simulink library "sm_trackV_lib_chain_segment"  (R2026a)
settings: Solver=VariableStepAuto
undefined symbols (not defined in the file): Excv, X, Y, Z
libraries: sm_lib x43, $bdroot x10
(part 2 of 2)

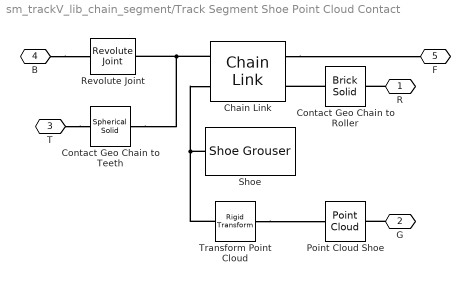
== system sm_trackV_lib_chain_segment/Track Segment Shoe Point Cloud Contact ==
  Chain Link : $bdroot/Chain Link  chain_wid=chain_wid  chain_seg_m=chain_seg_m  chain_seg_cg=chain_seg_cg  chain_seg_moi=chain_seg_moi  chain_seg_poi=chain_seg_poi  plate_h=plate_h  plate_xc=plate_xc  plate_thk=plate_thk  pin_sep=pin_sep  plate_ang=plate_ang  plate_clr=plate_clr  plate_opc=plate_opc  pin_len=pin_len  pin_rad=pin_rad  pin_clr=pin_clr  pin_opc=pin_opc
  Contact Geo Chain to Roller : sm_lib/Body Elements/Brick Solid  BrickDimensions=[pin_sep plate_h chain_wid/2]  BrickDimensionsUnits=m  ExportEntireGeometry=on  InertiaType=CalculateFromGeometry  BasedOnType=Density  Density=0  DensityUnits=kg/m^3  Mass=1  MassUnits=kg  CenterOfMass=[0 0 0]  CenterOfMassUnits=m  MomentsOfInertia=[1 1 1]  MomentsOfInertiaUnits=kg*m^2  ProductsOfInertia=[0 0 0]  ProductsOfInertiaUnits=kg*m^2  GraphicType=FromGeometry  MarkerShape=Sphere  MarkerSize=10  GraphicVisPropType=SimpleVisualProperties  GraphicDiffuseColor=chain_to_roller_clr  GraphicOpacity=chain_to_roller_opc  GraphicSpecularColor=[0.5 0.5 0.5 1.0]  GraphicAmbientColor=[0.15 0.15 0.15 1.0]  GraphicEmissiveColor=[0.0 0.0 0.0 1.0]  GraphicShininess=75  DoExposeReferenceFrame=on  SerializedFrames=<Frames/>
  Contact Geo Chain to Teeth : sm_lib/Body Elements/Spherical Solid  SphereRadius=pin_rad  SphereRadiusUnits=m  ExportEntireGeometry=on  InertiaType=CalculateFromGeometry  BasedOnType=Density  Density=0  DensityUnits=kg/m^3  Mass=1  MassUnits=kg  CenterOfMass=[0 0 0]  CenterOfMassUnits=m  MomentsOfInertia=[1 1 1]  MomentsOfInertiaUnits=kg*m^2  ProductsOfInertia=[0 0 0]  ProductsOfInertiaUnits=kg*m^2  GraphicType=FromGeometry  MarkerShape=Sphere  MarkerSize=10  GraphicVisPropType=SimpleVisualProperties  GraphicDiffuseColor=chain_to_teeth_clr  GraphicOpacity=chain_to_teeth_opc  GraphicSpecularColor=[0.5 0.5 0.5 1.0]  GraphicAmbientColor=[0.15 0.15 0.15 1.0]  GraphicEmissiveColor=[0.0 0.0 0.0 1.0]  GraphicShininess=75  DoExposeReferenceFrame=on  SerializedFrames=<Frames/>
  Point Cloud Shoe : sm_lib/Curves and Surfaces/Point Cloud  CoordinatesMatrix=ptcld_shoe  CoordinatesMatrixUnits=m  GraphicType=MarkerCloud  GraphicSphereRadius=ptcld_shoe_rad  GraphicSphereRadiusUnits=m  GraphicVisPropType=SimpleVisualProperties  GraphicDiffuseColor=ptcld_shoe_clr  GraphicOpacity=ptcld_shoe_opc  GraphicSpecularColor=[0.5 0.5 0.5 1.0]  GraphicAmbientColor=[0.15 0.15 0.15 1.0]  GraphicEmissiveColor=[0.0 0.0 0.0 1.0]  GraphicShininess=75
  Revolute Joint : sm_lib/Joints/Revolute Joint  JointMode=Normal  CompositeWrenchDir=FollowerOnBase  CompositeWrenchFrame=BaseFrame  SenseConstraintForce=off  SenseConstraintTorque=off  SenseTotalForce=off  SenseTotalTorque=off  PositionTargetSpecify=on  PositionTargetPriority=High  PositionTargetValue=PositionTargetValue  PositionTargetValueUnits=deg  VelocityTargetSpecify=off  VelocityTargetPriority=High  VelocityTargetValue=0  VelocityTargetValueUnits=deg/s  EquilibriumPosition=0  EquilibriumPositionUnits=deg  SpringStiffness=0  SpringStiffnessUnits=N*m/deg  DampingCoefficient=DampingCoefficient  DampingCoefficientUnits=N*m/(deg/s)  LowerLimitSpecify=off  LowerLimitBound=-10  LowerLimitBoundUnits=deg  LowerLimitStiffness=1e2  LowerLimitStiffnessUnits=N*m/deg  LowerLimitDamping=10  LowerLimitDampingUnits=N*m/(deg/s)  LowerLimitTransitionRegionWidth=0.1  LowerLimitTransitionRegionWidthUnits=deg  UpperLimitSpecify=off  UpperLimitBound=65  UpperLimitBoundUnits=deg  UpperLimitStiffness=1e2  UpperLimitStiffnessUnits=N*m/deg  UpperLimitDamping=10  UpperLimitDampingUnits=N*m/(deg/s)  UpperLimitTransitionRegionWidth=0.1  UpperLimitTransitionRegionWidthUnits=deg  TorqueActuationMode=NoTorque  MotionActuationMode=ComputedMotion  SensePosition=off  SenseVelocity=off  SenseAcceleration=off  SenseTorqueForce=off  SenseLowerLimitTorqueForce=off  SenseUpperLimitTorqueForce=off
  Shoe : $bdroot/Shoe Grouser  shoe_xc=shoe_xc  shoe_w=shoe_w  shoe_m=shoe_m  shoe_cg=shoe_cg  shoe_moi=shoe_moi  shoe_poi=shoe_poi  shoe_clr=shoe_clr  shoe_opc=shoe_opc
      settings: LibrarySourceBlock=sm_chain_drive_lib/Shoe
  Transform Point Cloud : sm_lib/Frames and Transforms/Rigid Transform  RotationMethod=StandardAxis  FollAlignAxisA=+X  BaseAlignAxisA=+Y  FollAlignAxisB=+Y  BaseAlignAxisB=+Z  RotationStandardAxis=+Y  RotationAngle=180  RotationAngleUnits=deg  RotationArbitraryAxis=[0 0 1]  RotationSequenceAxes=FollowerAxes  RotationSequence=XYX  RotationSequenceAngles=[0 0 0]  RotationSequenceAnglesUnits=deg  RotationMatrix=[1 0 0; 0 1 0; 0 0 1]  Quaternion=[1 0 0 0]  TranslationMethod=None  TranslationCartesianOffset=[0 0 0]  TranslationCartesianOffsetUnits=m  TranslationStandardAxis=-Y  TranslationStandardOffset=0  TranslationStandardOffsetUnits=m  TranslationROffset=0  TranslationROffsetUnits=m  TranslationThetaOffset=0  TranslationThetaOffsetUnits=deg  TranslationZOffset=0  TranslationZOffsetUnits=m
  R : PMIOPort  Side=Right
  G : PMIOPort  Port=2  Side=Right
  T : PMIOPort  Port=3  Side=Right
  B : PMIOPort  Port=4  Side=Left
  F : PMIOPort  Port=5  Side=Left
  connections:
  Transform Point Cloud/RConn1 -- Point Cloud Shoe/LConn1
  Contact Geo Chain to Teeth/RConn1 -- Chain Link/RConn1 -- Revolute Joint/LConn1
  Shoe/RConn1 -- Transform Point Cloud/LConn1 -- Chain Link/RConn2
  B/RConn1 -- Revolute Joint/RConn1
  G/RConn1 -- Point Cloud Shoe/RConn1
  T/RConn1 -- Contact Geo Chain to Teeth/LConn1
  Contact Geo Chain to Roller/RConn1 -- Chain Link/LConn2
  R/RConn1 -- Contact Geo Chain to Roller/LConn1
  Chain Link/LConn1 -- F/RConn1

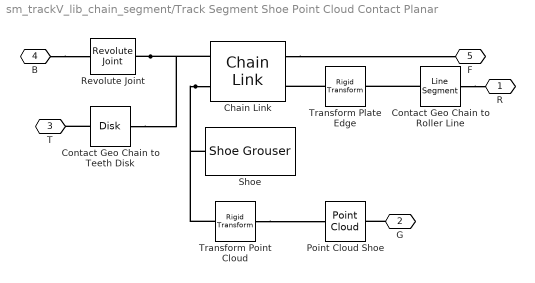
== system sm_trackV_lib_chain_segment/Track Segment Shoe Point Cloud Contact Planar ==
  Chain Link : $bdroot/Chain Link  chain_wid=chain_wid  chain_seg_m=chain_seg_m  chain_seg_cg=chain_seg_cg  chain_seg_moi=chain_seg_moi  chain_seg_poi=chain_seg_poi  plate_h=plate_h  plate_xc=plate_xc  plate_thk=plate_thk  pin_sep=pin_sep  plate_ang=plate_ang  plate_clr=plate_clr  plate_opc=plate_opc  pin_len=pin_len  pin_rad=pin_rad  pin_clr=pin_clr  pin_opc=pin_opc
  Contact Geo Chain to Roller Line : sm_lib/Curves and Surfaces/Line Segment  Length=pin_sep  LengthUnits=m  GraphicType=FromGeometry  GraphicVisPropType=SimpleVisualProperties  GraphicDiffuseColor=chain_to_roller_clr  GraphicOpacity=chain_to_roller_opc  GraphicSpecularColor=[0.5 0.5 0.5 1.0]  GraphicAmbientColor=[0.15 0.15 0.15 1.0]  GraphicEmissiveColor=[0.0 0.0 0.0 1.0]  GraphicShininess=75
  Contact Geo Chain to Teeth Disk : sm_lib/Curves and Surfaces/Disk  Radius=pin_rad  RadiusUnits=m  GraphicType=FromGeometry  GraphicVisPropType=SimpleVisualProperties  GraphicDiffuseColor=chain_to_teeth_clr  GraphicOpacity=chain_to_teeth_opc  GraphicSpecularColor=[0.5 0.5 0.5 1.0]  GraphicAmbientColor=[0.15 0.15 0.15 1.0]  GraphicEmissiveColor=[0.0 0.0 0.0 1.0]  GraphicShininess=75
  Point Cloud Shoe : sm_lib/Curves and Surfaces/Point Cloud  CoordinatesMatrix=ptcld_shoe  CoordinatesMatrixUnits=m  GraphicType=MarkerCloud  GraphicSphereRadius=ptcld_shoe_rad  GraphicSphereRadiusUnits=m  GraphicVisPropType=SimpleVisualProperties  GraphicDiffuseColor=ptcld_shoe_clr  GraphicOpacity=ptcld_shoe_opc  GraphicSpecularColor=[0.5 0.5 0.5 1.0]  GraphicAmbientColor=[0.15 0.15 0.15 1.0]  GraphicEmissiveColor=[0.0 0.0 0.0 1.0]  GraphicShininess=75
  Revolute Joint : sm_lib/Joints/Revolute Joint  JointMode=Normal  CompositeWrenchDir=FollowerOnBase  CompositeWrenchFrame=BaseFrame  SenseConstraintForce=off  SenseConstraintTorque=off  SenseTotalForce=off  SenseTotalTorque=off  PositionTargetSpecify=on  PositionTargetPriority=High  PositionTargetValue=PositionTargetValue  PositionTargetValueUnits=deg  VelocityTargetSpecify=off  VelocityTargetPriority=High  VelocityTargetValue=0  VelocityTargetValueUnits=deg/s  EquilibriumPosition=0  EquilibriumPositionUnits=deg  SpringStiffness=0  SpringStiffnessUnits=N*m/deg  DampingCoefficient=DampingCoefficient  DampingCoefficientUnits=N*m/(deg/s)  LowerLimitSpecify=off  LowerLimitBound=-10  LowerLimitBoundUnits=deg  LowerLimitStiffness=1e2  LowerLimitStiffnessUnits=N*m/deg  LowerLimitDamping=10  LowerLimitDampingUnits=N*m/(deg/s)  LowerLimitTransitionRegionWidth=0.1  LowerLimitTransitionRegionWidthUnits=deg  UpperLimitSpecify=off  UpperLimitBound=65  UpperLimitBoundUnits=deg  UpperLimitStiffness=1e2  UpperLimitStiffnessUnits=N*m/deg  UpperLimitDamping=10  UpperLimitDampingUnits=N*m/(deg/s)  UpperLimitTransitionRegionWidth=0.1  UpperLimitTransitionRegionWidthUnits=deg  TorqueActuationMode=NoTorque  MotionActuationMode=ComputedMotion  SensePosition=off  SenseVelocity=off  SenseAcceleration=off  SenseTorqueForce=off  SenseLowerLimitTorqueForce=off  SenseUpperLimitTorqueForce=off
  Shoe : $bdroot/Shoe Grouser  shoe_xc=shoe_xc  shoe_w=shoe_w  shoe_m=shoe_m  shoe_cg=shoe_cg  shoe_moi=shoe_moi  shoe_poi=shoe_poi  shoe_clr=shoe_clr  shoe_opc=shoe_opc
      settings: LibrarySourceBlock=sm_chain_drive_lib/Shoe
  Transform Plate Edge : sm_lib/Frames and Transforms/Rigid Transform  RotationMethod=None  FollAlignAxisA=+X  BaseAlignAxisA=+Y  FollAlignAxisB=+Y  BaseAlignAxisB=+Z  RotationStandardAxis=+Z  RotationAngle=0.0  RotationAngleUnits=deg  RotationArbitraryAxis=[0 0 1]  RotationSequenceAxes=FollowerAxes  RotationSequence=XYX  RotationSequenceAngles=[0 0 0]  RotationSequenceAnglesUnits=deg  RotationMatrix=[1 0 0; 0 1 0; 0 0 1]  Quaternion=[1 0 0 0]  TranslationMethod=StandardAxis  TranslationCartesianOffset=[0 0 0]  TranslationCartesianOffsetUnits=m  TranslationStandardAxis=+Y  TranslationStandardOffset=plate_h/2  TranslationStandardOffsetUnits=m  TranslationROffset=0  TranslationROffsetUnits=m  TranslationThetaOffset=0  TranslationThetaOffsetUnits=deg  TranslationZOffset=0  TranslationZOffsetUnits=m
  Transform Point Cloud : sm_lib/Frames and Transforms/Rigid Transform  RotationMethod=StandardAxis  FollAlignAxisA=+X  BaseAlignAxisA=+Y  FollAlignAxisB=+Y  BaseAlignAxisB=+Z  RotationStandardAxis=+Y  RotationAngle=180  RotationAngleUnits=deg  RotationArbitraryAxis=[0 0 1]  RotationSequenceAxes=FollowerAxes  RotationSequence=XYX  RotationSequenceAngles=[0 0 0]  RotationSequenceAnglesUnits=deg  RotationMatrix=[1 0 0; 0 1 0; 0 0 1]  Quaternion=[1 0 0 0]  TranslationMethod=None  TranslationCartesianOffset=[0 0 0]  TranslationCartesianOffsetUnits=m  TranslationStandardAxis=-Y  TranslationStandardOffset=0  TranslationStandardOffsetUnits=m  TranslationROffset=0  TranslationROffsetUnits=m  TranslationThetaOffset=0  TranslationThetaOffsetUnits=deg  TranslationZOffset=0  TranslationZOffsetUnits=m
  R : PMIOPort  Side=Right
  G : PMIOPort  Port=2  Side=Right
  T : PMIOPort  Port=3  Side=Right
  B : PMIOPort  Port=4  Side=Left
  F : PMIOPort  Port=5  Side=Left
  connections:
  Contact Geo Chain to Roller Line/LConn1 -- Transform Plate Edge/RConn1
  Chain Link/LConn1 -- F/RConn1
  Contact Geo Chain to Roller Line/RConn1 -- R/RConn1
  Transform Plate Edge/LConn1 -- Chain Link/LConn2
  Contact Geo Chain to Teeth Disk/RConn1 -- T/RConn1
  G/RConn1 -- Point Cloud Shoe/RConn1
  B/RConn1 -- Revolute Joint/RConn1
  Chain Link/RConn2 -- Transform Point Cloud/LConn1 -- Shoe/RConn1
  Revolute Joint/LConn1 -- Contact Geo Chain to Teeth Disk/LConn1 -- Chain Link/RConn1
  Transform Point Cloud/RConn1 -- Point Cloud Shoe/LConn1

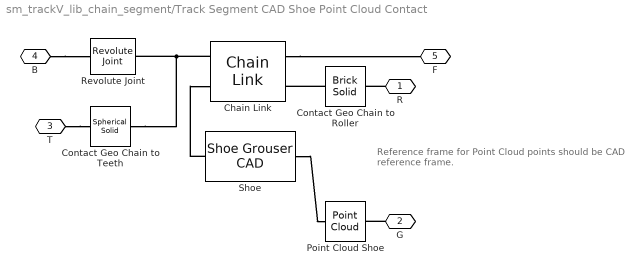
== system sm_trackV_lib_chain_segment/Track Segment CAD Shoe Point Cloud Contact ==
  note: Reference frame for Point Cloud points should be CAD reference frame.
  Chain Link : $bdroot/Chain Link  chain_wid=chain_wid  chain_seg_m=chain_seg_m  chain_seg_cg=chain_seg_cg  chain_seg_moi=chain_seg_moi  chain_seg_poi=chain_seg_poi  plate_h=plate_h  plate_xc=plate_xc  plate_thk=plate_thk  pin_sep=pin_sep  plate_ang=plate_ang  plate_clr=plate_clr  plate_opc=plate_opc  pin_len=pin_len  pin_rad=pin_rad  pin_clr=pin_clr  pin_opc=pin_opc
  Contact Geo Chain to Roller : sm_lib/Body Elements/Brick Solid  BrickDimensions=[pin_sep plate_h chain_wid/2]  BrickDimensionsUnits=m  ExportEntireGeometry=on  InertiaType=CalculateFromGeometry  BasedOnType=Density  Density=0  DensityUnits=kg/m^3  Mass=1  MassUnits=kg  CenterOfMass=[0 0 0]  CenterOfMassUnits=m  MomentsOfInertia=[1 1 1]  MomentsOfInertiaUnits=kg*m^2  ProductsOfInertia=[0 0 0]  ProductsOfInertiaUnits=kg*m^2  GraphicType=FromGeometry  MarkerShape=Sphere  MarkerSize=10  GraphicVisPropType=SimpleVisualProperties  GraphicDiffuseColor=chain_to_roller_clr  GraphicOpacity=chain_to_roller_opc  GraphicSpecularColor=[0.5 0.5 0.5 1.0]  GraphicAmbientColor=[0.15 0.15 0.15 1.0]  GraphicEmissiveColor=[0.0 0.0 0.0 1.0]  GraphicShininess=75  DoExposeReferenceFrame=on  SerializedFrames=<Frames/>
  Contact Geo Chain to Teeth : sm_lib/Body Elements/Spherical Solid  SphereRadius=pin_rad  SphereRadiusUnits=m  ExportEntireGeometry=on  InertiaType=CalculateFromGeometry  BasedOnType=Density  Density=0  DensityUnits=kg/m^3  Mass=1  MassUnits=kg  CenterOfMass=[0 0 0]  CenterOfMassUnits=m  MomentsOfInertia=[1 1 1]  MomentsOfInertiaUnits=kg*m^2  ProductsOfInertia=[0 0 0]  ProductsOfInertiaUnits=kg*m^2  GraphicType=FromGeometry  MarkerShape=Sphere  MarkerSize=10  GraphicVisPropType=SimpleVisualProperties  GraphicDiffuseColor=chain_to_teeth_clr  GraphicOpacity=chain_to_teeth_opc  GraphicSpecularColor=[0.5 0.5 0.5 1.0]  GraphicAmbientColor=[0.15 0.15 0.15 1.0]  GraphicEmissiveColor=[0.0 0.0 0.0 1.0]  GraphicShininess=75  DoExposeReferenceFrame=on  SerializedFrames=<Frames/>
  Point Cloud Shoe : sm_lib/Curves and Surfaces/Point Cloud  CoordinatesMatrix=ptcld_shoe  CoordinatesMatrixUnits=m  GraphicType=MarkerCloud  GraphicSphereRadius=ptcld_shoe_rad  GraphicSphereRadiusUnits=m  GraphicVisPropType=SimpleVisualProperties  GraphicDiffuseColor=ptcld_shoe_clr  GraphicOpacity=ptcld_shoe_opc  GraphicSpecularColor=[0.5 0.5 0.5 1.0]  GraphicAmbientColor=[0.15 0.15 0.15 1.0]  GraphicEmissiveColor=[0.0 0.0 0.0 1.0]  GraphicShininess=75
  Revolute Joint : sm_lib/Joints/Revolute Joint  JointMode=Normal  CompositeWrenchDir=FollowerOnBase  CompositeWrenchFrame=BaseFrame  SenseConstraintForce=off  SenseConstraintTorque=off  SenseTotalForce=off  SenseTotalTorque=off  PositionTargetSpecify=on  PositionTargetPriority=High  PositionTargetValue=PositionTargetValue  PositionTargetValueUnits=deg  VelocityTargetSpecify=off  VelocityTargetPriority=High  VelocityTargetValue=0  VelocityTargetValueUnits=deg/s  EquilibriumPosition=0  EquilibriumPositionUnits=deg  SpringStiffness=0  SpringStiffnessUnits=N*m/deg  DampingCoefficient=DampingCoefficient  DampingCoefficientUnits=N*m/(deg/s)  LowerLimitSpecify=off  LowerLimitBound=-10  LowerLimitBoundUnits=deg  LowerLimitStiffness=1e2  LowerLimitStiffnessUnits=N*m/deg  LowerLimitDamping=10  LowerLimitDampingUnits=N*m/(deg/s)  LowerLimitTransitionRegionWidth=0.1  LowerLimitTransitionRegionWidthUnits=deg  UpperLimitSpecify=off  UpperLimitBound=65  UpperLimitBoundUnits=deg  UpperLimitStiffness=1e2  UpperLimitStiffnessUnits=N*m/deg  UpperLimitDamping=10  UpperLimitDampingUnits=N*m/(deg/s)  UpperLimitTransitionRegionWidth=0.1  UpperLimitTransitionRegionWidthUnits=deg  TorqueActuationMode=NoTorque  MotionActuationMode=ComputedMotion  SensePosition=off  SenseVelocity=off  SenseAcceleration=off  SenseTorqueForce=off  SenseLowerLimitTorqueForce=off  SenseUpperLimitTorqueForce=off
  Shoe : $bdroot/Shoe Grouser CAD  shoe_xc=shoe_xc  shoe_w=shoe_w  shoe_m=shoe_m  shoe_cg=shoe_cg  shoe_moi=shoe_moi  shoe_poi=shoe_poi  shoe_clr=shoe_clr  shoe_opc=shoe_opc
  R : PMIOPort  Side=Right
  G : PMIOPort  Port=2  Side=Right
  T : PMIOPort  Port=3  Side=Right
  B : PMIOPort  Port=4  Side=Left
  F : PMIOPort  Port=5  Side=Left
  connections:
  Shoe/LConn1 -- Point Cloud Shoe/LConn1
  Contact Geo Chain to Teeth/RConn1 -- Chain Link/RConn1 -- Revolute Joint/LConn1
  Shoe/RConn1 -- Chain Link/RConn2
  B/RConn1 -- Revolute Joint/RConn1
  G/RConn1 -- Point Cloud Shoe/RConn1
  T/RConn1 -- Contact Geo Chain to Teeth/LConn1
  Contact Geo Chain to Roller/RConn1 -- Chain Link/LConn2
  R/RConn1 -- Contact Geo Chain to Roller/LConn1
  Chain Link/LConn1 -- F/RConn1

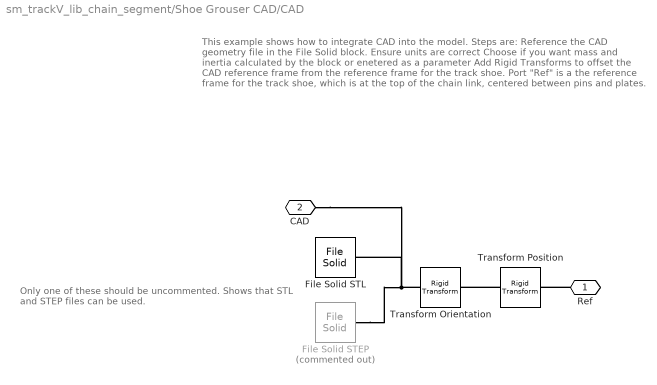
== system sm_trackV_lib_chain_segment/Shoe Grouser CAD/CAD ==
  note: This example shows how to integrate CAD into the model.
      | Steps are:
      | Reference the CAD geometry file in the File Solid block.
      | Ensure units are correct
      | Choose if you want mass and inertia calculated by the block or enetered as a parameter
      | Add Rigid Transforms to offset the CAD reference frame from the reference frame for the track shoe.
      | Port "Ref" is a the reference frame for the track shoe, which is at the top of the chain link, centered between pins and plates.
  note: Only one of these should be uncommented. Shows that STL and STEP files can be used.
  File Solid STEP : sm_lib/Body Elements/File Solid  Commented=on  ExtGeomFileName=CAD_Track_Shoe.STEP  UnitType=FromFile  ExtGeomFileUnits=mm  StepReaderType=HEX  ExportConvexHullGeometry=off  InertiaType=PointMass  BasedOnType=Density  Density=2700  DensityUnits=kg/m^3  Mass=0  MassUnits=kg  CenterOfMass=[0 0 0]  CenterOfMassUnits=m  MomentsOfInertia=[1 1 1]  MomentsOfInertiaUnits=kg*m^2  ProductsOfInertia=[0 0 0]  ProductsOfInertiaUnits=kg*m^2  GraphicType=FromGeometry  MarkerShape=Sphere  MarkerSize=10  GraphicVisPropType=SimpleVisualProperties  GraphicDiffuseColor=shoe_clr  GraphicOpacity=shoe_opc  GraphicSpecularColor=[0.5 0.5 0.5 1.0]  GraphicAmbientColor=[0.15 0.15 0.15 1.0]  GraphicEmissiveColor=[0.0 0.0 0.0 1.0]  GraphicShininess=75  DoExposeReferenceFrame=on  SerializedFrames=<Frames/>
  File Solid STL : sm_lib/Body Elements/File Solid  ExtGeomFileName=CAD_Track_Shoe.STL  UnitType=Custom  ExtGeomFileUnits=mm  StepReaderType=HEX  ExportConvexHullGeometry=off  InertiaType=PointMass  BasedOnType=Density  Density=2700  DensityUnits=kg/m^3  Mass=0  MassUnits=kg  CenterOfMass=[0 0 0]  CenterOfMassUnits=m  MomentsOfInertia=[1 1 1]  MomentsOfInertiaUnits=kg*m^2  ProductsOfInertia=[0 0 0]  ProductsOfInertiaUnits=kg*m^2  GraphicType=FromGeometry  MarkerShape=Sphere  MarkerSize=10  GraphicVisPropType=SimpleVisualProperties  GraphicDiffuseColor=shoe_clr  GraphicOpacity=shoe_opc  GraphicSpecularColor=[0.5 0.5 0.5 1.0]  GraphicAmbientColor=[0.15 0.15 0.15 1.0]  GraphicEmissiveColor=[0.0 0.0 0.0 1.0]  GraphicShininess=75  DoExposeReferenceFrame=on  SerializedFrames=<Frames/>
  Transform Orientation : sm_lib/Frames and Transforms/Rigid Transform  RotationMethod=StandardAxis  FollAlignAxisA=+X  BaseAlignAxisA=+Y  FollAlignAxisB=+Y  BaseAlignAxisB=+Z  RotationStandardAxis=+Z  RotationAngle=180  RotationAngleUnits=deg  RotationArbitraryAxis=[0 0 1]  RotationSequenceAxes=FollowerAxes  RotationSequence=XYX  RotationSequenceAngles=[0 0 0]  RotationSequenceAnglesUnits=deg  RotationMatrix=[1 0 0; 0 1 0; 0 0 1]  Quaternion=[1 0 0 0]  TranslationMethod=None  TranslationCartesianOffset=[0 0 0]  TranslationCartesianOffsetUnits=m  TranslationStandardAxis=+Z  TranslationStandardOffset=0  TranslationStandardOffsetUnits=m  TranslationROffset=0  TranslationROffsetUnits=m  TranslationThetaOffset=0  TranslationThetaOffsetUnits=deg  TranslationZOffset=0  TranslationZOffsetUnits=m
  Transform Position : sm_lib/Frames and Transforms/Rigid Transform  RotationMethod=None  FollAlignAxisA=+X  BaseAlignAxisA=+Y  FollAlignAxisB=+Y  BaseAlignAxisB=+Z  RotationStandardAxis=+Z  RotationAngle=0.0  RotationAngleUnits=deg  RotationArbitraryAxis=[0 0 1]  RotationSequenceAxes=FollowerAxes  RotationSequence=XYX  RotationSequenceAngles=[0 0 0]  RotationSequenceAnglesUnits=deg  RotationMatrix=[1 0 0; 0 1 0; 0 0 1]  Quaternion=[1 0 0 0]  TranslationMethod=StandardAxis  TranslationCartesianOffset=[0 0 0]  TranslationCartesianOffsetUnits=m  TranslationStandardAxis=+Z  TranslationStandardOffset=0.3  TranslationStandardOffsetUnits=m  TranslationROffset=0  TranslationROffsetUnits=m  TranslationThetaOffset=0  TranslationThetaOffsetUnits=deg  TranslationZOffset=0  TranslationZOffsetUnits=m
  Ref : PMIOPort  Side=Right
  CAD : PMIOPort  Port=2  Side=Left
  connections:
  Ref/RConn1 -- Transform Position/RConn1
  CAD/RConn1 -- File Solid STL/RConn1 -- File Solid STEP/RConn1 -- Transform Orientation/LConn1
  Transform Position/LConn1 -- Transform Orientation/RConn1
